simulink model "BatchingExperiment_2016a"  (R2016a)
settings: Solver=VariableStepAuto  StartTime=0.0  StopTime=100  FixedStep=1  RelTol=1e-3
undefined symbols (not defined in the file): m, n
settings Model: Creator=tsprock3  LastModifiedBy=tsprock3

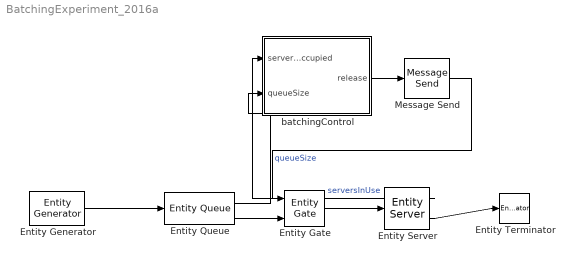
== system BatchingExperiment_2016a ==
  Entity Gate : EntityGate  InputPortMessageModes=m,m  OutputPortMessageModes=m
  Entity Generator : EntityGenerator  OutputPortMessageModes=m  EntityType=Structured  EntityTypeName=Entity
  Entity Queue : EntityQueue  InputPortMessageModes=m  OutputPortMessageModes=n,m  NumberEntitiesInBlock=on
      settings: OutputPortMap=o1,o5
  Entity Server : EntityServer  InputPortMessageModes=m  OutputPortMessageModes=n,m  ServiceTimeValue=5  NumberEntitiesInBlock=on
      settings: OutputPortMap=o1,o9
  Entity Terminator : EntityTerminator  InputPortMessageModes=m
  Message Send : MessageSend  OutputPortMessageModes=m
      settings: InputPortMap=u1
  batchingControl : Stateflow chart  TreatAsAtomicUnit=on
  wires:
  Entity Queue/2 -> Entity Gate/2
  Entity Gate/1 -> Entity Server/1
  Entity Server/1 -> batchingControl/1(serverOccupied)  "serversInUse"
  Entity Queue/1 -> batchingControl/2(queueSize)  "queueSize"
  Entity Generator/1 -> Entity Queue/1
  Entity Server/2 -> Entity Terminator/1
  batchingControl/1(release) -> Message Send/1
  Message Send/1 -> Entity Gate/1

== stateflow chart BatchingExperiment_2016a/batchingControl ==
  settings: updateMethod=DISCRETE  sampleTime=0.5
  state IncompleteBatch
    entry:
    release = 0;
  state Processing
    entry:
    release = 0;
  state CompleteBatch
    entry:
    release =1;
  (default) -> IncompleteBatch
  Processing -> IncompleteBatch : [serverOccupied == 0]
  IncompleteBatch -> CompleteBatch : [queueSize >=5]
  CompleteBatch -> Processing : [serverOccupied == 5]
  data: serverOccupied input; queueSize input; release output
